simulink model "a_present"  (R2013a)
settings: Solver=ode45  StartTime=0.0  StopTime=10000  RelTol=1e-3
settings Model: Creator=Leo  LastModifiedBy=Leo

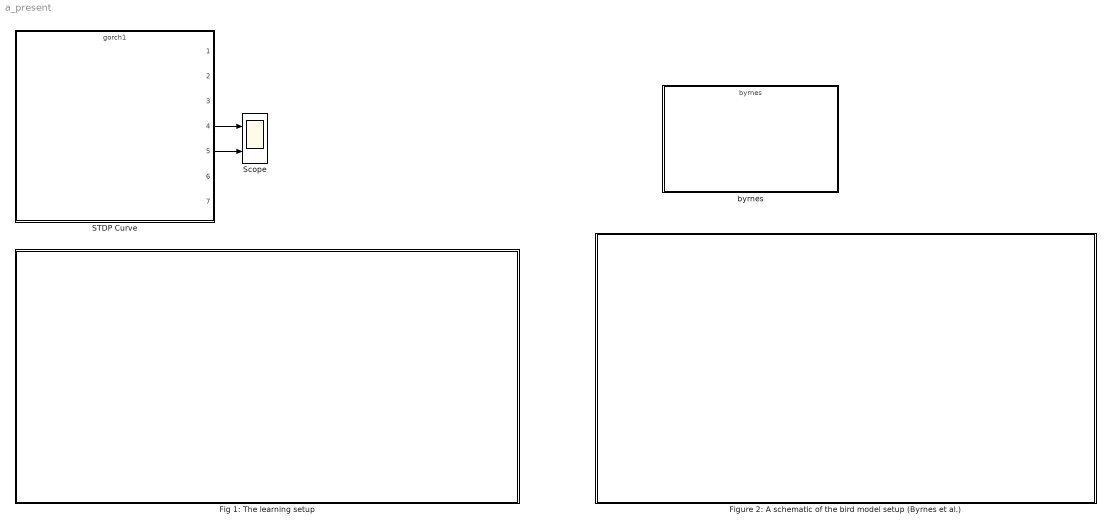
== system a_present ==
  Fig 1: The learning setup : Subsystem
      mask Display: image(imread('pic1.png'));
  Figure 2: A schematic of the bird model setup (Byrnes et al.) : Subsystem
      mask Display: image(imread('pic2.png'));
  STDP Curve : ModelReference  ModelNameDialog=gorch1.mdl  SimulationMode=Normal  ModelReferenceVersion=1.482  CopyOfModelName=gorch1.mdl  DefaultDataLogging=off
  Scope : Scope  NumInputPorts=2
      settings: TimeRange=1000  YMin=-60~-0.4  YMax=140~1
  byrnes : ModelReference  ModelNameDialog=byrnes.mdl  SimulationMode=Normal  ModelReferenceVersion=1.23  CopyOfModelName=byrnes.mdl  DefaultDataLogging=on
  wires:
  STDP Curve/4 -> Scope/1
  STDP Curve/5 -> Scope/2

== system a_present/Fig 1: The learning setup ==

== system a_present/Figure 2: A schematic of the bird model setup (Byrnes et al.) ==
